simulink model "single_phase_pwm_rectifier_closeloop"  (R2022b)
settings: Solver=VariableStepAuto  StartTime=0.0  StopTime=1  FixedStep=1e-6  MaxStep=1e-8  RelTol=1e-7
model workspace (MAT data in the model file):
  Kp = 1
  Kr = 10
  Ts = 2.5e-05
  wc = 6.28318530718
  wr = 314.159265359
undefined symbols (not defined in the file): DiscIntNeverNeededParam, sigbuilder_block
libraries: spsMosfetLib x4, dspsigops x3, spsSeriesRLCBranchLib x3, simulink x2, slpidlib x2, spsVoltageMeasurementLib x2, spsACVoltageSourceLib x1, spsCurrentMeasurementLib x1, spsIdealSwitchLib x1, eeGeneralControl x1, spspowerguiLib x1
settings Model: Creator=SSC  LastModifiedBy=SSC

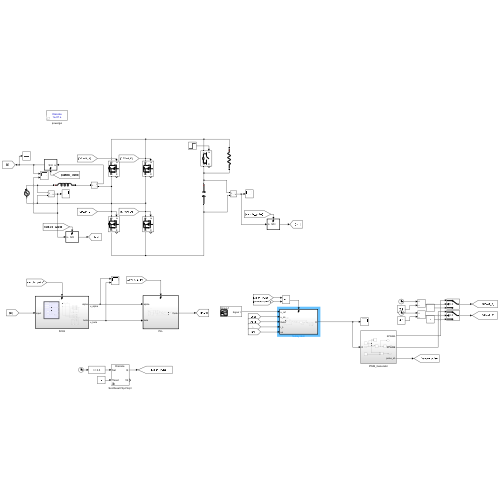
[thumbnail: Simulink's stored preview of the top-level diagram]
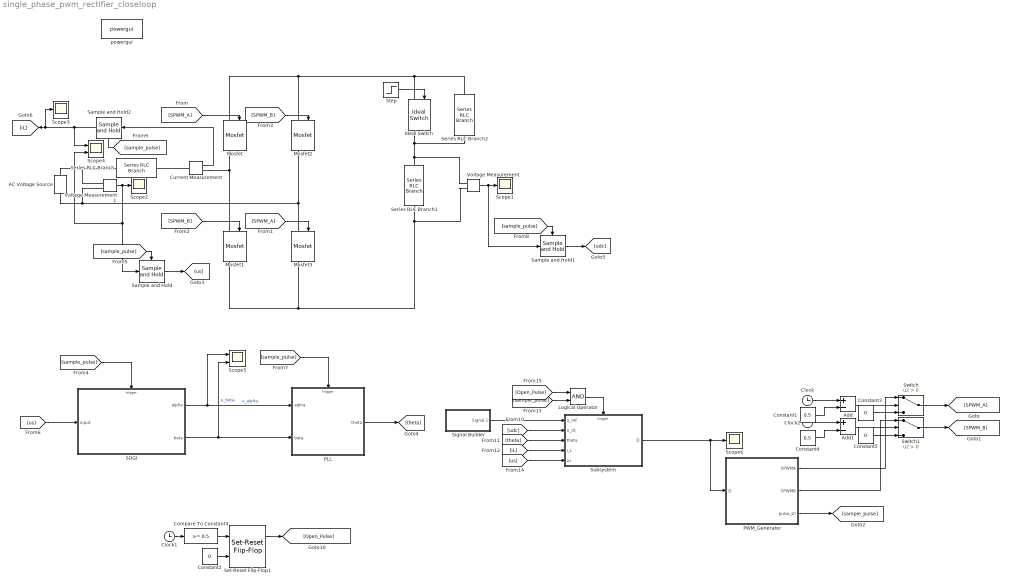
== system single_phase_pwm_rectifier_closeloop ==
  AC Voltage Source : spsACVoltageSourceLib/AC Voltage Source  Amplitude=24*sqrt(2)  Phase=0  Frequency=50  SampleTime=0  Measurements=Voltage  BusType=swing  Pref=10e3  Qref=0  Qmin=-inf  Qmax=+inf
  Add : Sum  Inputs=+-
  Add1 : Sum  Inputs=+-
  Clock : Clock
  Clock1 : Clock
  Clock2 : Clock
  Compare To Constant4 : simulink/Logic and Bit Operations/Compare To Constant  relop=>=  const=0.5  OutDataTypeStr=boolean
  Constant1 : Constant  Value=0.5
  Constant2 : Constant  Value=0
  Constant3 : Constant  Value=0
  Constant4 : Constant  Value=0.5
  Constant5 : Constant  Value=0
  Current Measurement : spsCurrentMeasurementLib/Current Measurement  PhasorSimulation=off  OutputType=Complex  PSBequivalent=0
  Ideal Switch : spsIdealSwitchLib/Ideal Switch  Ron=0.001  Lon=0  IC=0  Rs=1e5  Cs=inf  Measurements=on
  Logical Operator : Logic  AllPortsSameDT=off  OutDataTypeStr=boolean
  Mosfet{,1..3} (4 alike) : spsMosfetLib/Mosfet  Ron=0.1  Lon=0  Rd=0.01  Vfd=0  IC=0  Rs=1e5  Cs=inf  Measurements=on
  PLL : Subsystem  TreatAsAtomicUnit=on
  PWM_Generator : Subsystem
  SOGI : Subsystem  TreatAsAtomicUnit=on
  Sample and Hold : dspsigops/Sample and Hold  trig=Rising edge  initCond=0  latchinput=off
  Sample and Hold1 : dspsigops/Sample and Hold  trig=Rising edge  initCond=0  latchinput=off
  Sample and Hold2 : dspsigops/Sample and Hold  trig=Rising edge  initCond=0  latchinput=off
  Scope{1..3,6} (4 alike) : Scope
  Scope4 : Scope  NumInputPorts=2
  Scope5 : Scope  NumInputPorts=2
  Series RLC Branch : spsSeriesRLCBranchLib/Series RLC Branch  LConnTagsString=__new0  RConnTagsString=__new0  BranchType=L  Resistance=1  Inductance=2e-3  SetiL0=off  InitialCurrent=0  Capacitance=1e-6  Setx0=off  InitialVoltage=0  Measurements=Branch voltage and current
  Series RLC Branch1 : spsSeriesRLCBranchLib/Series RLC Branch  LConnTagsString=__new0  RConnTagsString=__new0  BranchType=C  Resistance=1  Inductance=1e-3  SetiL0=off  InitialCurrent=0  Capacitance=3*1200e-6  Setx0=off  InitialVoltage=0  Measurements=None
  Series RLC Branch2 : spsSeriesRLCBranchLib/Series RLC Branch  LConnTagsString=__new0  RConnTagsString=__new0  BranchType=R  Resistance=12  Inductance=1e-3  SetiL0=off  InitialCurrent=0  Capacitance=3*1200e-6  Setx0=off  InitialVoltage=0  Measurements=None
  Set-Reset Flip-Flop1 : eeGeneralControl/Set-Reset Flip-Flop  LabelModeActiveChoice=Discrete  UndefState=Set  Q0=0  Ts=-1
      settings: LibrarySourceBlock=ee_sl_lib/General Control/Set-Reset Flip-Flop
  Signal Builder : Subsystem  Tag=STV Subsys  LoadFcn=sigbuilder_block('load');  StartFcn=sigbuilder_block('start');  StopFcn=sigbuilder_block('stop');  ClipboardFcn=sigbuilder_block('clipboard');  mask(Sigbuilder block){tuvar=[0:10]}
      mask help: Simulink:masks:SigbuilderBlock_MD
      mask init:
      | if ~strcmp(get_param(bdroot(gcbh),'SimulationStatus'),'stopped') tuvar = sigbuilder_block('maskInit'); end
      settings: CopyFcn=sigbuilder_block('copy');  DeleteFcn=sigbuilder_block('delete');  ModelCloseFcn=sigbuilder_block('modelClose');  PreSaveFcn=sigbuilder_block('preSave');  PauseFcn=sigbuilder_block('pause');  ContinueFcn=sigbuilder_block('continue');  NameChangeFcn=sigbuilder_block('namechange');  OpenFcn=sigbuilder_block('open',[6 36 1428 674.25 ]);  CloseFcn=sigbuilder_block('close');
      mask Display: plot(0, 0, 100, 100,[2, 2, 32, 32, 2], [68, 8, 8, 68, 68],[32, 2], [38, 38], [32, 19, 2],[53, 60, 44], [32, 17, 17, 2],[16, 16, 31, 31]);txt = getActiveGroup(gcbh);text(2, 100, txt,'verticalAlignment', 'top');
  Step : Step  Time=0.5  SampleTime=0
  Subsystem : Subsystem
  Switch : Switch  Criteria=u2 > Threshold  SaturateOnIntegerOverflow=off  InputSameDT=off
  Switch1 : Switch  Criteria=u2 > Threshold  SaturateOnIntegerOverflow=off  InputSameDT=off
  Voltage Measurement : spsVoltageMeasurementLib/Voltage Measurement  PhasorSimulation=off  OutputType=Complex  PSBequivalent=0
  Voltage Measurement1 : spsVoltageMeasurementLib/Voltage Measurement  PhasorSimulation=off  OutputType=Complex  PSBequivalent=0
  powergui : spspowerguiLib/powergui  Priority=1  SimulationMode=Discrete  SampleTime=1e-7  frequency=60  Iterations=50  frequencyindice=0  Pbase=100e6  ErrMax=1e-4  UnitsV=kV  UnitsW=MW  buscounter=0  FunctionMessages=off  echomessages=off  EnableUseOfTLC=off  CurrentSourceSwitches=off  DisableSnubberDevices=off  DisableRonSwitches=off  DisableVfSwitches=off  DisplayEquations=off  AutomaticDiscreteSolvers=off  SolverType=Tustin/Backward Euler (TBE)  Interpol=off  ExternalGateDelay=off  methode=off  Ts=100  x0status=blocks  SPID=on  SwTol=0  HookPort=off  NonlinearTolerance=1e-4  nMaxIteration=100  ContinueOnMaxIteration=off  RestoreLinks=warning  ResistiveCurrentMeasurement=off  Frange=[0:2:500]  Ylog=off  Xlog=on  ShowGrid=off  save=off  variable=ZData  structure=0  ZoomFFT=off  StartTime=0.0  cycles=1  DisplayStyle=1  fundamental=60  FreqAxis=off  MaxFrequency=1000  frequencyindicesteady=1  RmsSteady=1  display=off
  wires:
  PWM_Generator/3(pulse_sh) -> [sample_pulse]
  [sample_pulse] -> SOGI/Trigger
  [us] -> SOGI/1(input)
  SOGI/1(alpha) -> PLL/1(alpha), Scope5/1  "u_alpha"
  SOGI/2(beta) -> PLL/2(beta), Scope5/2  "u_beta"
  [sample_pulse] -> PLL/Trigger
  PLL/1(theta) -> [theta]
  [udc] -> Subsystem/2(u_dc)
  Signal Builder/1(Signal 1) -> Subsystem/1(u_ref)
  [theta] -> Subsystem/3(theta)
  [iL] -> Subsystem/4(i_L)
  [SPWM_B] -> Mosfet1/1
  [SPWM_B] -> Mosfet2/1
  [SPWM_A] -> Mosfet3/1
  [SPWM_A] -> Mosfet/1
  Voltage Measurement1/1 -> Scope4/2, Sample and Hold/1, Scope2/1
  [sample_pulse] -> Sample and Hold/Trigger
  Sample and Hold/1 -> [us]
  [sample_pulse] -> Sample and Hold1/Trigger
  Voltage Measurement/1 -> Sample and Hold1/1, Scope1/1
  Sample and Hold1/1 -> [udc]
  [sample_pulse] -> Sample and Hold2/Trigger
  Current Measurement/1 -> Sample and Hold2/1
  [us] -> Subsystem/5(us)
  Sample and Hold2/1 -> Scope3/1, [iL], Scope4/1
  Clock/1 -> Add/1
  Add/1 -> Switch/2
  Constant1/1 -> Add/2
  Constant2/1 -> Set-Reset Flip-Flop1/2
  Compare To Constant4/1 -> Set-Reset Flip-Flop1/1
  Set-Reset Flip-Flop1/1 -> [Open_Pulse]
  Clock1/1 -> Compare To Constant4/1
  [sample_pulse] -> Logical Operator/2
  Logical Operator/1 -> Subsystem/Trigger
  [Open_Pulse] -> Logical Operator/1
  Constant3/1 -> Switch/3
  Subsystem/1(D) -> PWM_Generator/1(D), Scope6/1
  PWM_Generator/1(SPWMA) -> Switch/1
  Switch/1 -> [SPWM_A]
  Switch1/1 -> [SPWM_B]
  Constant5/1 -> Switch1/3
  Constant4/1 -> Add1/2
  PWM_Generator/2(SPWMB) -> Switch1/1
  Clock2/1 -> Add1/1
  Add1/1 -> Switch1/2
  Step/1 -> Ideal Switch/1
  connections:
  Series RLC Branch1/LConn1 -- Series RLC Branch2/RConn1 -- Ideal Switch/RConn1 -- Voltage Measurement/LConn1
  Voltage Measurement/LConn2 -- Mosfet3/RConn1 -- Mosfet1/RConn1 -- Series RLC Branch1/RConn1
  Mosfet3/LConn1 -- Voltage Measurement1/LConn2 -- AC Voltage Source/LConn1 -- Mosfet2/RConn1
  Series RLC Branch/LConn1 -- Voltage Measurement1/LConn1 -- AC Voltage Source/RConn1
  Mosfet/RConn1 -- Current Measurement/RConn1 -- Mosfet1/LConn1
  Current Measurement/LConn1 -- Series RLC Branch/RConn1
  Mosfet/LConn1 -- Series RLC Branch2/LConn1 -- Ideal Switch/LConn1 -- Mosfet2/LConn1

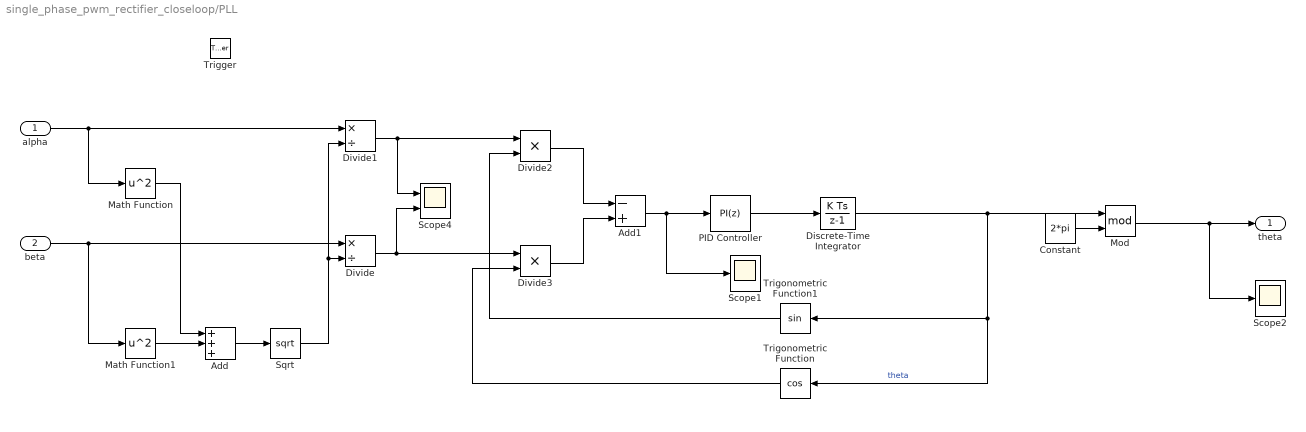
== system single_phase_pwm_rectifier_closeloop/PLL ==
  alpha : Inport
  beta : Inport  Port=2
  Trigger : TriggerPort  VariantControl=(inherit)
  Add : Sum  Inputs=+++
  Add1 : Sum  Inputs=-+
  Constant : Constant  Value=2*pi
  Discrete-Time Integrator : DiscreteIntegrator  SampleTime=-1  ICPrevOutput=DiscIntNeverNeededParam  ICPrevScaledInput=DiscIntNeverNeededParam
  Divide : Product  Inputs=*/
  Divide1 : Product  Inputs=*/
  Divide2 : Product  Inputs=**
  Divide3 : Product  Inputs=**
  Math Function : Math  Operator=square
  Math Function1 : Math  Operator=square
  Mod : Math  Operator=mod
  PID Controller : slpidlib/PID Controller  Controller=PI  Form=Parallel  TimeDomain=Discrete-time  UseExternalTs=off  SampleTime=-1  IntegratorMethod=Forward Euler  FilterMethod=Forward Euler  ControllerParametersSource=internal  P=5000  I=2000000  UseKiTs=off  D=0  N=100  UseFilter=on  TunerSelectOption=Transfer Function Based (PID Tuner App)  InitialConditionSource=internal  InitialConditionForIntegrator=0  InitialConditionForFilter=0  DifferentiatorICPrevScaledInput=0  ExternalReset=none  TrackingMode=off  Kt=1  LimitOutput=off  SatLimitsSource=internal  UpperSaturationLimit=inf  LowerSaturationLimit=-inf  LinearizeAsGain=on  AntiWindupMode=none  Kb=1  LimitIntegrator=off  UpperIntegratorSaturationLimit=inf  LowerIntegratorSaturationLimit=-inf  POutMin=[]  POutMax=[]  IOutMin=[]  IOutMax=[]  DOutMin=[]  DOutMax=[]  NOutMin=[]  NOutMax=[]  SumOutMin=[]  SumOutMax=[]  SaturationOutMin=[]  SaturationOutMax=[]  PParamMin=[]  PParamMax=[]  IParamMin=[]  IParamMax=[]  DParamMin=[]  DParamMax=[]  NParamMin=[]  NParamMax=[]  KbParamMin=[]  KbParamMax=[]  KtParamMin=[]  KtParamMax=[]  KbOutMin=[]  KbOutMax=[]  KtOutMin=[]  KtOutMax=[]  IntegratorOutMin=[]  IntegratorOutMax=[]  FilterOutMin=[]  FilterOutMax=[]  SumI1OutMin=[]  SumI1OutMax=[]  SumI2OutMin=[]  SumI2OutMax=[]  SumI3OutMin=[]  SumI3OutMax=[]  SumI4OutMin=[]  SumI4OutMax=[]  SumDOutMin=[]  SumDOutMax=[]  DifferentiatorOutMin=[]  DifferentiatorOutMax=[]  FilterDiffOutCoefMin=[]  FilterDiffOutCoefMax=[]  ReciprocalOutMin=[]  ReciprocalOutMax=[]  SumDenOutMin=[]  SumDenOutMax=[]  SumNumOutMin=[]  SumNumOutMax=[]  DivideOutMin=[]  DivideOutMax=[]  UdiffTsProdOutMin=[]  UdiffTsProdOutMax=[]  NTsProdOutMin=[]  NTsProdOutMax=[]  UintegralTsProdOutMin=[]  UintegralTsProdOutMax=[]  UngainTsProdOutMin=[]  UngainTsProdOutMax=[]  ClampingZeroOutDataTypeStr=Inherit: Inherit via back propagation  ClampingZeroOutMin=[]  ClampingZeroOutMax=[]  FilterDenConstantOutDataTypeStr=Inherit: Inherit via back propagation  FilterDenConstantOutMin=[]  FilterDenConstantOutMax=[]  PCopyOutDataTypeStr=Inherit: Inherit via back propagation  PCopyOutMin=[]  PCopyOutMax=[]  NCopyOutDataTypeStr=Inherit: Inherit via back propagation  NCopyOutMin=[]  NCopyOutMax=[]  IntegratorContinuousStateAttributes=''  IntegratorStateMustResolveToSignalObject=off  IntegratorRTWStateStorageClass=Auto  FilterContinuousStateAttributes=''  FilterStateMustResolveToSignalObject=off  FilterRTWStateStorageClass=Auto  ParallelPVariant=InternalParameters  IdealPVariant=Disabled  IVariant=InternalParameters  DVariant=Disabled  IntegratorVariant=Discrete  SatVariant=Disabled  AWVariant=Passthrough  PCopyVariant=Disabled  TRVariant=Disabled  FdbkBlocksVariant=Forward  IdealPFdbkVariant=Disabled  SatFdbkVariant=Disabled  DerivativeFilterVariant=Disabled  NVariant=Disabled  NCopyVariant=Disabled_SignalSpec  FilterICVariant=Disabled  IntegratorICVariant=InternalICs  ExternalResetVariant=Disabled  TRSumVariant=Passthrough  SumFdbkVariant=Disabled  SumVariant=Sum_PI  TsampFilterVariant=InternalTs  TsampNgainVariant=Passthrough  TsampIntegralVariant=Passthrough  ExternalSaturationOutDataTypeStr=Inherit: Same as second input
  Scope1 : Scope
  Scope2 : Scope
  Scope4 : Scope  NumInputPorts=2
  Sqrt : Sqrt
  Trigonometric Function : Trigonometry  Operator=cos
  Trigonometric Function1 : Trigonometry
  theta : Outport
  wires:
  alpha/1 -> Divide1/1, Math Function/1
  beta/1 -> Divide/1, Math Function1/1
  Math Function1/1 -> Add/2
  Math Function/1 -> Add/1
  Add/1 -> Sqrt/1
  Divide1/1 -> Scope4/1, Divide2/1
  Divide/1 -> Scope4/2, Divide3/1
  Divide2/1 -> Add1/1
  Divide3/1 -> Add1/2
  Add1/1 -> Scope1/1, PID Controller/1
  PID Controller/1 -> Discrete-Time Integrator/1
  Discrete-Time Integrator/1 -> Mod/1, Trigonometric Function/1, Trigonometric Function1/1  "theta"
  Trigonometric Function1/1 -> Divide2/2
  Trigonometric Function/1 -> Divide3/2
  Sqrt/1 -> Divide1/2, Divide/2
  Constant/1 -> Mod/2
  Mod/1 -> Scope2/1, theta/1

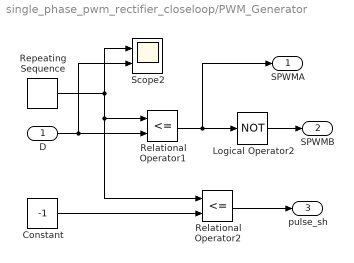
== system single_phase_pwm_rectifier_closeloop/PWM_Generator ==
  D : Inport
  Constant : Constant  Value=-1
  Logical Operator2 : Logic  Operator=NOT  AllPortsSameDT=off  OutDataTypeStr=boolean
  Relational Operator1 : RelationalOperator  Operator=<=  OutDataTypeStr=boolean  RndMeth=Simplest  InputSameDT=off
  Relational Operator2 : RelationalOperator  Operator=<=  OutDataTypeStr=boolean  RndMeth=Simplest  InputSameDT=off
  Repeating Sequence : simulink/Sources/Repeating Sequence  rep_seq_t=[0 0.125e-4 0.25e-4]  rep_seq_y=[-1 1 -1]
  Scope2 : Scope  NumInputPorts=2
  SPWMA : Outport
  SPWMB : Outport  Port=2
  pulse_sh : Outport  Port=3
  wires:
  Relational Operator1/1 -> SPWMA/1, Logical Operator2/1
  Logical Operator2/1 -> SPWMB/1
  D/1 -> Scope2/2, Relational Operator1/2
  Repeating Sequence/1 -> Relational Operator2/1, Relational Operator1/1, Scope2/1
  Relational Operator2/1 -> pulse_sh/1
  Constant/1 -> Relational Operator2/2

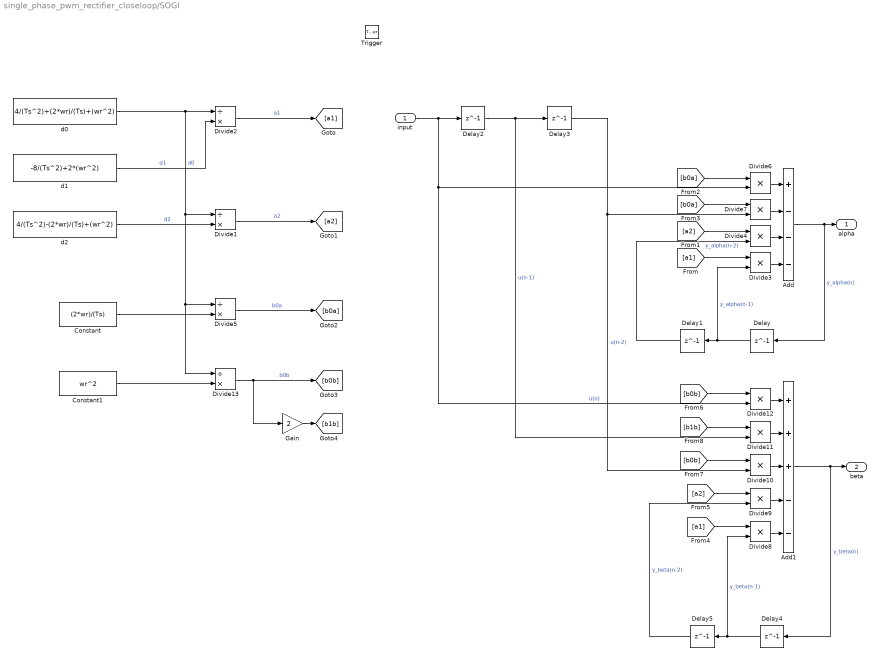
== system single_phase_pwm_rectifier_closeloop/SOGI ==
  input : Inport
  Trigger : TriggerPort  VariantControl=(inherit)
  Add : Sum  Inputs=+---
  Add1 : Sum  Inputs=+++--
  Constant : Constant  Value=(2*wr)/(Ts)
  Constant1 : Constant  Value=wr^2
  Delay{,1..5} (6 alike) : Delay  DelayLength=1  InitialCondition=0
  Divide{1..2,5,13} (4 alike) : Product  Inputs=/*
  Divide{3..4,6..12} (9 alike) : Product  Inputs=**
  Gain : Gain  Gain=2
  d0 : Constant  Value=4/(Ts^2)+(2*wr)/(Ts)+(wr^2)
  d1 : Constant  Value=-8/(Ts^2)+2*(wr^2)
  d2 : Constant  Value=4/(Ts^2)-(2*wr)/(Ts)+(wr^2)
  alpha : Outport
  beta : Outport  Port=2
  wires:
  d0/1 -> Divide2/1, Divide5/1, Divide13/1, Divide1/1  "d0"
  d1/1 -> Divide2/2  "d1"
  d2/1 -> Divide1/2  "d2"
  Divide2/1 -> [a1]  "a1"
  Divide1/1 -> [a2]  "a2"
  Add/1 -> Delay/1, alpha/1  "y_alpha(n)"
  Delay/1 -> Divide3/2, Delay1/1  "y_alpha(n-1)"
  Delay1/1 -> Divide4/2  "y_alpha(n-2)"
  Divide3/1 -> Add/4
  [a1] -> Divide3/1
  Divide4/1 -> Add/3
  [a2] -> Divide4/1
  Divide5/1 -> [b0a]  "b0a"
  Constant/1 -> Divide5/2
  Divide6/1 -> Add/1
  [b0a] -> Divide6/1
  Divide7/1 -> Add/2
  input/1 -> Divide12/2, Divide6/2, Delay2/1  "u(n)"
  Delay2/1 -> Divide11/2, Delay3/1  "u(n-1)"
  Delay3/1 -> Divide10/2, Divide7/2  "u(n-2)"
  [b0a] -> Divide7/1
  Add1/1 -> Delay4/1, beta/1  "y_beta(n)"
  Delay5/1 -> Divide9/2  "y_beta(n-2)"
  Delay4/1 -> Divide8/2, Delay5/1  "y_beta(n-1)"
  Divide8/1 -> Add1/5
  [a1] -> Divide8/1
  Divide9/1 -> Add1/4
  [a2] -> Divide9/1
  Divide10/1 -> Add1/3
  Divide11/1 -> Add1/2
  Divide12/1 -> Add1/1
  Constant1/1 -> Divide13/2
  Divide13/1 -> Gain/1, [b0b]  "b0b"
  Gain/1 -> [b1b]
  [b0b] -> Divide12/1
  [b0b] -> Divide10/1
  [b1b] -> Divide11/1

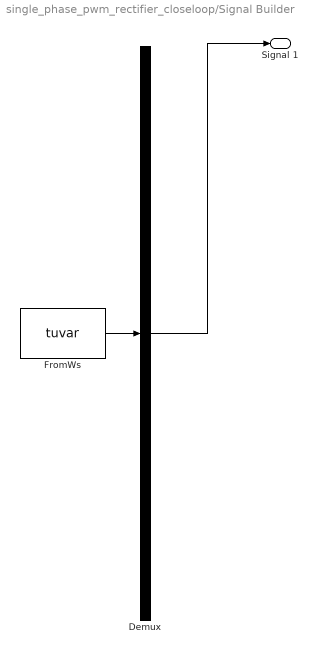
== system single_phase_pwm_rectifier_closeloop/Signal Builder ==
  Demux : Demux  Tag=STV Demux  Outputs=1
      settings: DisplayOption=none
  FromWs : FromWorkspace  Tag=STV FromWs  VariableName=tuvar
      SigBuilderData=|
      | common.afterFinalStr = 'Extrapolate'
      | common.sampleTime = 0
      | dataSet.timeRange = [0 13]
      | dataSet.name = 'Group 1'
      | sbobj.Groups.Name = 'Group 1'
      | sbobj.Groups.Signals.Name = 'Signal 1'
      | sbobj.Groups.Signals.XData = [0 0.5 0.8 13]
      | sbobj.Groups.Signals.YData = [30 30 50 50]
      | sbobj.Groups.TimeRange = [0 13]
  Signal 1 : Outport  Tag=STV Outport
  wires:
  Demux/1 -> Signal 1/1
  FromWs/1 -> Demux/1

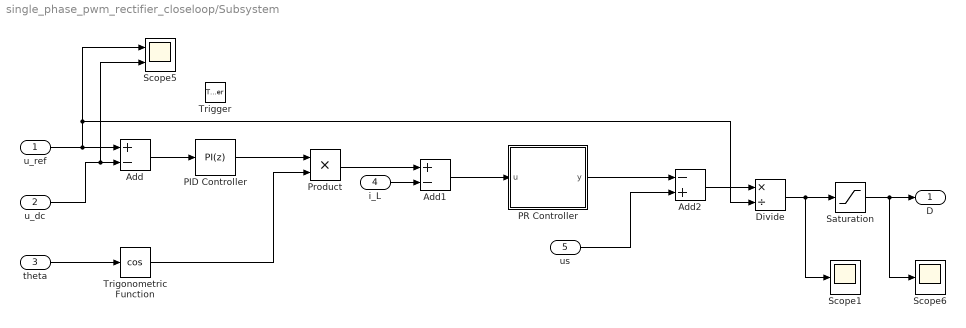
== system single_phase_pwm_rectifier_closeloop/Subsystem ==
  u_ref : Inport
  u_dc : Inport  Port=2
  theta : Inport  Port=3
  i_L : Inport  Port=4
  us : Inport  Port=5
  Trigger : TriggerPort  VariantControl=(inherit)  PortDimensions=1
  Add : Sum  Inputs=+-
  Add1 : Sum  Inputs=+-
  Add2 : Sum  Inputs=-+
  Divide : Product  Inputs=*/
  PID Controller : slpidlib/PID Controller  Controller=PI  Form=Parallel  TimeDomain=Discrete-time  UseExternalTs=off  SampleTime=-1  IntegratorMethod=Forward Euler  FilterMethod=Forward Euler  ControllerParametersSource=internal  P=0.8  I=10  UseKiTs=off  D=0  N=100  UseFilter=on  TunerSelectOption=Transfer Function Based (PID Tuner App)  InitialConditionSource=internal  InitialConditionForIntegrator=0  InitialConditionForFilter=0  DifferentiatorICPrevScaledInput=0  ExternalReset=none  TrackingMode=off  Kt=1  LimitOutput=off  SatLimitsSource=internal  UpperSaturationLimit=inf  LowerSaturationLimit=-inf  LinearizeAsGain=on  AntiWindupMode=none  Kb=1  LimitIntegrator=off  UpperIntegratorSaturationLimit=inf  LowerIntegratorSaturationLimit=-inf  POutMin=[]  POutMax=[]  IOutMin=[]  IOutMax=[]  DOutMin=[]  DOutMax=[]  NOutMin=[]  NOutMax=[]  SumOutMin=[]  SumOutMax=[]  SaturationOutMin=[]  SaturationOutMax=[]  PParamMin=[]  PParamMax=[]  IParamMin=[]  IParamMax=[]  DParamMin=[]  DParamMax=[]  NParamMin=[]  NParamMax=[]  KbParamMin=[]  KbParamMax=[]  KtParamMin=[]  KtParamMax=[]  KbOutMin=[]  KbOutMax=[]  KtOutMin=[]  KtOutMax=[]  IntegratorOutMin=[]  IntegratorOutMax=[]  FilterOutMin=[]  FilterOutMax=[]  SumI1OutMin=[]  SumI1OutMax=[]  SumI2OutMin=[]  SumI2OutMax=[]  SumI3OutMin=[]  SumI3OutMax=[]  SumI4OutMin=[]  SumI4OutMax=[]  SumDOutMin=[]  SumDOutMax=[]  DifferentiatorOutMin=[]  DifferentiatorOutMax=[]  FilterDiffOutCoefMin=[]  FilterDiffOutCoefMax=[]  ReciprocalOutMin=[]  ReciprocalOutMax=[]  SumDenOutMin=[]  SumDenOutMax=[]  SumNumOutMin=[]  SumNumOutMax=[]  DivideOutMin=[]  DivideOutMax=[]  UdiffTsProdOutMin=[]  UdiffTsProdOutMax=[]  NTsProdOutMin=[]  NTsProdOutMax=[]  UintegralTsProdOutMin=[]  UintegralTsProdOutMax=[]  UngainTsProdOutMin=[]  UngainTsProdOutMax=[]  ClampingZeroOutDataTypeStr=Inherit: Inherit via back propagation  ClampingZeroOutMin=[]  ClampingZeroOutMax=[]  FilterDenConstantOutDataTypeStr=Inherit: Inherit via back propagation  FilterDenConstantOutMin=[]  FilterDenConstantOutMax=[]  PCopyOutDataTypeStr=Inherit: Inherit via back propagation  PCopyOutMin=[]  PCopyOutMax=[]  NCopyOutDataTypeStr=Inherit: Inherit via back propagation  NCopyOutMin=[]  NCopyOutMax=[]  IntegratorContinuousStateAttributes=''  IntegratorStateMustResolveToSignalObject=off  IntegratorRTWStateStorageClass=Auto  FilterContinuousStateAttributes=''  FilterStateMustResolveToSignalObject=off  FilterRTWStateStorageClass=Auto  ParallelPVariant=InternalParameters  IdealPVariant=Disabled  IVariant=InternalParameters  DVariant=Disabled  IntegratorVariant=Discrete  SatVariant=Disabled  AWVariant=Passthrough  PCopyVariant=Disabled  TRVariant=Disabled  FdbkBlocksVariant=Forward  IdealPFdbkVariant=Disabled  SatFdbkVariant=Disabled  DerivativeFilterVariant=Disabled  NVariant=Disabled  NCopyVariant=Disabled_SignalSpec  FilterICVariant=Disabled  IntegratorICVariant=InternalICs  ExternalResetVariant=Disabled  TRSumVariant=Passthrough  SumFdbkVariant=Disabled  SumVariant=Sum_PI  TsampFilterVariant=InternalTs  TsampNgainVariant=Passthrough  TsampIntegralVariant=Passthrough  ExternalSaturationOutDataTypeStr=Inherit: Same as second input
  PR Controller : Subsystem
  Product : Product
  Saturation : Saturate  UpperLimit=1  LowerLimit=-1
  Scope1 : Scope
  Scope5 : Scope  NumInputPorts=2
  Scope6 : Scope
  Trigonometric Function : Trigonometry  Operator=cos
  D : Outport
  wires:
  PID Controller/1 -> Product/1
  Add/1 -> PID Controller/1
  u_ref/1 -> Scope5/1, Divide/2, Add/1
  u_dc/1 -> Scope5/2, Add/2
  theta/1 -> Trigonometric Function/1
  Trigonometric Function/1 -> Product/2
  Product/1 -> Add1/1
  i_L/1 -> Add1/2
  Add1/1 -> PR Controller/1(u)
  PR Controller/1(y) -> Add2/1
  us/1 -> Add2/2
  Add2/1 -> Divide/1
  Saturation/1 -> Scope6/1, D/1
  Divide/1 -> Scope1/1, Saturation/1

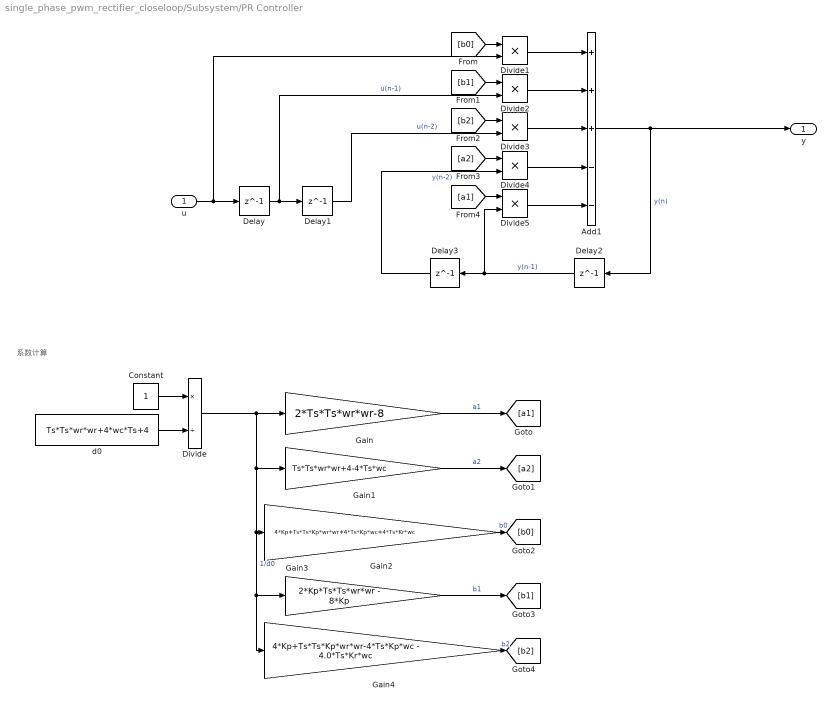
== system single_phase_pwm_rectifier_closeloop/Subsystem/PR Controller ==
  note: 系数计算
  u : Inport
  Add1 : Sum  Inputs=+++--
  Constant : Constant
  Delay{,1..3} (4 alike) : Delay  DelayLength=1  InitialCondition=0
  Divide : Product  Inputs=*/
  Divide{1..5} (5 alike) : Product  Inputs=**
  Gain : Gain  Gain=2*Ts*Ts*wr*wr-8
  Gain1 : Gain  Gain=Ts*Ts*wr*wr+4-4*Ts*wc
  Gain2 : Gain  Gain=4*Kp+Ts*Ts*Kp*wr*wr+4*Ts*Kp*wc+4*Ts*Kr*wc
  Gain3 : Gain  Gain=2*Kp*Ts*Ts*wr*wr - 8*Kp
  Gain4 : Gain  Gain=4*Kp+Ts*Ts*Kp*wr*wr-4*Ts*Kp*wc - 4.0*Ts*Kr*wc
  d0 : Constant  Value=Ts*Ts*wr*wr+4*wc*Ts+4
  y : Outport
  wires:
  u/1 -> Delay/1, Divide1/2
  Constant/1 -> Divide/1
  d0/1 -> Divide/2
  Divide/1 -> Gain4/1, Gain3/1, Gain2/1, Gain1/1, Gain/1  "1/d0"
  Gain/1 -> [a1]  "a1"
  Gain1/1 -> [a2]  "a2"
  Gain2/1 -> [b0]  "b0"
  Gain3/1 -> [b1]  "b1"
  Gain4/1 -> [b2]  "b2"
  Divide1/1 -> Add1/1
  [b0] -> Divide1/1
  Delay/1 -> Delay1/1, Divide2/2  "u(n-1)"
  Delay1/1 -> Divide3/2  "u(n-2)"
  [b1] -> Divide2/1
  [b2] -> Divide3/1
  Divide2/1 -> Add1/2
  Divide3/1 -> Add1/3
  Add1/1 -> y/1, Delay2/1  "y(n)"
  Delay2/1 -> Delay3/1, Divide5/2  "y(n-1)"
  Delay3/1 -> Divide4/2  "y(n-2)"
  Divide4/1 -> Add1/4
  Divide5/1 -> Add1/5
  [a2] -> Divide4/1
  [a1] -> Divide5/1
